simulink library "tqd"  (R2021b)
settings: Solver=VariableStepAuto  StartTime=0.0  StopTime=10.0  RelTol=1e-3
undefined symbols (not defined in the file or in its folder): ATQD_APSDecReq_X_kph, ATQD_APSDecReq_Y_mps2, ATQD_APSDecReqCMD_X_kph, ATQD_APSDecReqTs_X_pct, ATQD_APSDecTimeGain_X_Deg, ATQD_APSDecTimeGain_Y_s, ATQD_APSReqLowSpd_X_Deg, ATQD_AutoHoldReleaseBPS_X_Deg, ATQD_AWDLoadTrqnsGain_X_kg, ATQD_AWDLoadTrqnsGain_Y_pct, ATQD_BOSEnBPSPosn_X_kph, ATQD_BOSMap_X_rpm, ATQD_BOSMap_Y_pct, ATQD_CreepBaseTqD_X_kph, ATQD_CreepBaseTqD_Y_Deg, ATQD_CreepBaseTqR_X_kph, ATQD_CreepBaseTqR_Y_Deg, ATQD_CreepBPSDisPosn_X_Deg, ATQD_CreepBPSDisPosnR_X_Deg, ATQD_CreepBPSEnPosn_X_Deg, ATQD_CreepBPSEnPosnR_X_Deg, ATQD_CreepDeltaTq_X_kph, ATQD_CreepIterm_X_kph, ATQD_CreepIterm_Y_kph, ATQD_CreepItermMaxLimit_X_pct, ATQD_CreepPreloadTime_X_kph, ATQD_CreepPreloadTq_X_kph, ATQD_CreepPreloadTq_Y_s, ATQD_CreepProtTq_X_Deg, ATQD_CreepPterm_X_kph, ATQD_ECOTqMapD_X_rpm, ATQD_ECOTqMapD_Y_pct, ATQD_EOPDTqMapDCon_X_rpm, ATQD_EOPDTqMapDCon_Y_Deg, ATQD_EstInitVehWeight_X_c, ATQD_LHMRollGenMapD_X_rpm, ATQD_LHMRollGenMapD_Y_rpm, ATQD_LHMTqMapD_X_rpm, ATQD_LHMTqMapD_Y_pct, ATQD_NL1TqMapD_X_rpm, ATQD_NL1TqMapD_Y_pct, ATQD_NOPDTqMapDCon_X_rpm, ATQD_NOPDTqMapDCon_Y_Deg, ATQD_NRMRrEDUSpRat_X_rpm, ATQD_NRMRrEDUSpRat_Y_Nm, ATQD_OPDHoldDownRelDelay_X_Deg, ATQD_OPDHoldEnSpd_X_Deg, ATQD_OPDHoldRelDetTime_X_Deg, ATQD_OPDHoldReleaseTq_X_Deg, ATQD_OrigPedTqLowLim_X_Deg, ATQD_OrigPedTqLowLim_Y_pct, ATQD_PedalMapClimbUpLim_X_rpm, ATQD_PedalMapClimbUpLim_Y_Deg, ATQD_PreLoadTq_X_s, ATQD_RollGenMapEL1_X_rpm, ATQD_RollGenMapEL1_Y_rpm, ATQD_SL1TqMapD_X_rpm, ATQD_SL1TqMapD_Y_pct, ATQD_SlideRegenTqGain_X_Gps, ATQD_SlideRegenTqGain_Y_pct ... (+444)
libraries: hcu_lib x70, simulink x61, tqr x1
(part 6 of 14)

== system tqd/TQD/TorqueDemand/Signal_convert/RWDMCUReadyExt_flg ==
  VINP_RrMCUErr_enum : Inport
  Action Port : ActionPort
  Constant : Constant  Value=ENUM_MCUWARN_LV0
  Constant1 : Constant  Value=ENUM_MCUWARN_NOERROR
  Equal : RelationalOperator  Operator===  OutDataTypeStr=boolean  RndMeth=Simplest
  Equal1 : RelationalOperator  Operator===  OutDataTypeStr=boolean  RndMeth=Simplest
  Logical Operator : Logic  Operator=OR  AllPortsSameDT=off  OutDataTypeStr=boolean
  VTQD_RWDMCUReadyExt_flg : Outport
  wires:
  Logical Operator/1 -> VTQD_RWDMCUReadyExt_flg/1
  VINP_RrMCUErr_enum/1 -> Equal1/1, Equal/1
  Equal1/1 -> Logical Operator/2
  Equal/1 -> Logical Operator/1
  Constant1/1 -> Equal1/2
  Constant/1 -> Equal/2

== system tqd/TQD/TorqueDemand/Signal_convert/Regen Level Switch Botton ==
  task_time_s : Inport
  SWC_RegenUp : Inport  Port=2
  SWC_RegenDown : Inport  Port=3
  Constant13 : Constant  Value=ENUM_REGENSWSTA_SHORTPRESSUP
  Constant18 : Constant  Value=ENUM_REGENSWSTA_LONGPRESSUP
  Constant21 : Constant  Value=ENUM_REGENSWSTA_SHORTPRESSDOWN
  Constant23 : Constant  Value=ENUM_REGENSWSTA_LONGPRESSDOWN
  Constant24 : Constant  Value=ENUM_REGENSWSTA_NOACTION
  RegenDOWN : Subsystem
  RegenUP : Subsystem
  Switch{4,6..8} (4 alike) : Switch  Criteria=u2 ~= 0
  VTQD_RegenSWSta_enum : Outport
  wires:
  [SWC_RegenUP] -> RegenUP/2(SWC_RegenUp)
  Constant24/1 -> Switch8/3
  Constant13/1 -> Switch4/1
  [SWC_RegenDown] -> RegenDOWN/3(SWC_RegenDOWN)
  RegenDOWN/2(VTQD_RegenDownLongP_flg) -> Switch8/2
  Constant23/1 -> Switch8/1
  Constant21/1 -> Switch7/1
  Switch7/1 -> Switch6/3
  RegenDOWN/1(SWC_RegenDownShort_flg) -> Switch7/2
  [SWC_RegenUP] -> RegenDOWN/2(SWC_RegenUp)
  Constant18/1 -> Switch6/1
  RegenUP/2(VTQD_RegenUpLongP_flg) -> Switch6/2
  Switch6/1 -> Switch4/3
  RegenUP/1(SWC_RegenUpShort_flg) -> Switch4/2
  [SWC_RegenDown] -> RegenUP/3(SWC_RegenDOWN)
  SWC_RegenUp/1 -> [SWC_RegenUP]
  SWC_RegenDown/1 -> [SWC_RegenDown]
  Switch8/1 -> Switch7/3
  Switch4/1 -> VTQD_RegenSWSta_enum/1
  task_time_s/1 -> [task_time_s]
  [task_time_s] -> RegenUP/1(task_time_s)
  [task_time_s] -> RegenDOWN/1(task_time_s)

== system tqd/TQD/TorqueDemand/Signal_convert/SpdCtrlBotton Behavior ==
  note: If press time more then Long press's limit then go Long press only. Else go short press only. Else if no press.
  note: Long press or Short press
  SWC_ACC_Sta : Inport
  TASK_TIME : Inport  Port=2
  AND : Logic  AllPortsSameDT=off  OutDataTypeStr=boolean
  Constant10 : Constant  Value=FALSE
  Constant3 : Constant  Value=KTQD_SpdModeShortPLim_s
  Constant7 : Constant  Value=FALSE
  Default 3 sec : Constant  Value=KTQD_SpdModeLongPLim_s
  DelayEnable_LONG_PRESS : hcu_lib/Basic_Blocks/DelayEnable
  DelayEnable_SHORT_PRESS : hcu_lib/Basic_Blocks/DelayEnable
  Detect Decrease1 : simulink/Logic and Bit Operations/Detect Decrease  vinit=0.0  OutDataTypeStr=boolean
  Detect Decrease2 : simulink/Logic and Bit Operations/Detect Decrease  vinit=0.0  OutDataTypeStr=boolean
  Detect Increase : simulink/Logic and Bit Operations/Detect Increase  vinit=0.0  OutDataTypeStr=boolean
  Switch1 : Switch  Criteria=u2 > Threshold
  Switch2 : Switch  Criteria=u2 ~= 0
  VTQD_SpdCtrlShortP_flg : Outport
  "VTQD_SpdCtrlLongP_flg\t" : Outport  Port=2
  wires:
  Detect Increase/1 -> "VTQD_SpdCtrlLongP_flg\t"/1
  [TASK_TIME] -> DelayEnable_LONG_PRESS/3
  Default 3 sec/1 -> DelayEnable_LONG_PRESS/2
  [TASK_TIME] -> DelayEnable_SHORT_PRESS/3
  Constant3/1 -> DelayEnable_SHORT_PRESS/2
  DelayEnable_SHORT_PRESS/1 -> Detect Decrease2/1
  Constant7/1 -> Switch1/3
  DelayEnable_LONG_PRESS/1 -> Switch1/1, Switch1/2
  [Short_press_falling_Edge] -> AND/1
  [Long_press] -> Detect Decrease1/1, Detect Increase/1
  Constant10/1 -> Switch2/1
  [Short_press_falling_Edge] -> Switch2/3
  [SWC_ACC_Sta] -> DelayEnable_SHORT_PRESS/1, DelayEnable_LONG_PRESS/1
  AND/1 -> Switch2/2
  Switch2/1 -> VTQD_SpdCtrlShortP_flg/1
  SWC_ACC_Sta/1 -> [SWC_ACC_Sta]
  Detect Decrease1/1 -> AND/2
  Detect Decrease2/1 -> [Short_press_falling_Edge]
  Switch1/1 -> [Long_press]
  TASK_TIME/1 -> [TASK_TIME]

== system tqd/TQD/TorqueDemand/Signal_convert/Speed Setting Mode ==
  note: Botton logic
  note: INPUT Signal
  note: PWRSTA and DRIVE GEAR GOOD
  note: OUTPUT SET SPEED
  VPMM_PowerSta_enum : Inport
  VTQD_ShiftGearPosn_enum : Inport  Port=2
  VINP_VehSpeed_kph : Inport  Port=3
  VTQD_SpdCtrlMode_enum : Inport  Port=4
  VINP_ADASACCSta_enum : Inport  Port=5
  VVMC_CCCtrlSta_enum : Inport  Port=6
  VVMC_MSACtrlSta_enum : Inport  Port=7
  VINP_ADASVehSpdLim_kph : Inport  Port=8
  VTQD_SWCResUpSta_flg : Inport  Port=9
  VTQD_SWCSetDownSta_flg : Inport  Port=10
  VTQD_SWCCancelSta_flg : Inport  Port=11
  task_time_s : Inport  Port=12
  VVMC_LVDAACCStatusInformation_flg : Inport  Port=13
  VVMC_ACCObjDist_m : Inport  Port=14
  VVMC_MeterIndSpeed_raw32 : Inport  Port=15
  VINP_Distanceunit_flg : Inport  Port=16
  ACC Speed Setting ON : Subsystem  TreatAsAtomicUnit=on
  AND{1..5} (5 alike) : Logic  AllPortsSameDT=off  OutDataTypeStr=boolean
  CC Speed Setting ON : Subsystem  TreatAsAtomicUnit=on
  Constant : Constant  Value=ZERO_INT
  Constant1 : Constant  Value=ENUM_SPDCTRLMODE_CC
  Constant10 : Constant  Value=ENUM_SPDCTRLMODE_ISA
  Constant11 : Constant  Value=ENUM_SPDCTRLMODE_OFF
  Constant12 : Constant  Value=KTQD_SetSpdDeltaLongFit_kph
  Constant13 : Constant  Value=ZERO_INT
  Constant2 : Constant  Value=ENUM_POWERSTA_READY
  Constant3 : Constant  Value=ENUM_SPDCTRLMODE_ACC
  Constant4 : Constant  Value=ENUM_GEARPOSNTOCAN_D
  Constant5 : Constant  Value=ENUM_SPDCTRLMODE_MSA
  Constant6 : Constant  Value=ENUM_SPDCTRLMODE_ISA
  Constant7 : Constant  Value=ENUM_SPDCTRLMODE_ACC
  Constant8 : Constant  Value=ENUM_SPDCTRLMODE_CC
  Constant9 : Constant  Value=ENUM_SPDCTRLMODE_MSA
  Data Type Conversion : DataTypeConversion  OutDataTypeStr=uint8
  Delay : Delay  DelayLength=1
  Else Speed Setting On : Subsystem  TreatAsAtomicUnit=on
  Equal{1..11} (11 alike) : RelationalOperator  Operator===  OutDataTypeStr=boolean  RndMeth=Simplest
  ISA Speed Setting ON : Subsystem  TreatAsAtomicUnit=on
  If : If  NumInputs=4  IfExpression=u1 ~= 0  ElseIfExpressions=u2 ~= 0, u3~= 0, u4~= 0
  MSA Speed Setting ON : Subsystem  TreatAsAtomicUnit=on
  Rem : Math  Operator=rem  SaturateOnIntegerOverflow=on
  Switch{,1..4} (5 alike) : Switch  Criteria=u2 ~= 0
  VTQD_SWCCancelP_flg : Subsystem
  VTQD_SWCResUpPress_enum : Subsystem
  VTQD_SWCSetDownPress_enum : Subsystem
  VTQD_SetSpd_kph : Outport
  wires:
  MSA Speed Setting ON/1(VSCP_MSASetSpd_kph) -> [VTQD_MSASetSpd_kph]  "VTQD_MSASetSpd_kph"
  CC Speed Setting ON/1(VTQD_CCSetSpd_kph) -> [VTQD_CCSetSpd_kph]  "VTQD_CCSetSpd_kph"
  VVMC_CCCtrlSta_enum/1 -> [VVMC_CCCtrlSta_enum]
  VINP_ADASVehSpdLim_kph/1 -> [VINP_ADASVehSpdLim_kph]
  task_time_s/1 -> [task_time_s]
  Switch/1 -> [VTQD_SetSpd_kph], VTQD_SetSpd_kph/1
  Constant/1 -> Switch4/1
  Switch4/1 -> Switch3/3
  Equal11/1 -> Switch4/2
  [VTQD_SpdCtrlMode_enum] -> Equal11/1
  Constant11/1 -> Equal11/2
  Switch3/1 -> Switch2/3
  Constant10/1 -> Equal10/2
  [VTQD_SpdCtrlMode_enum] -> Equal10/1
  Equal10/1 -> Switch3/2
  [VTQD_ISASetSpd_kph] -> Switch3/1
  Switch2/1 -> Switch1/3
  [VTQD_MSASetSpd_kph] -> Switch2/1
  Equal9/1 -> Switch2/2
  [VTQD_SpdCtrlMode_enum] -> Equal9/1
  Constant9/1 -> Equal9/2
  Switch1/1 -> Switch/3
  Constant8/1 -> Equal8/2
  [VTQD_SpdCtrlMode_enum] -> Equal8/1
  Equal8/1 -> Switch1/2
  [VTQD_CCSetSpd_kph] -> Switch1/1
  [VTQD_ACCSetSpd_kph] -> Switch/1
  Equal7/1 -> Switch/2
  [VTQD_SpdCtrlMode_enum] -> Equal7/1
  Constant7/1 -> Equal7/2
  ISA Speed Setting ON/1(VTQD_ISASetSpd_kph) -> [VTQD_ISASetSpd_kph]  "VTQD_ISASetSpd_kph"
  If/5 -> Else Speed Setting On/Action
  If/4 -> ISA Speed Setting ON/Action
  AND5/1 -> If/4
  [VTQD_PwrstaANDGearGOOD_flg] -> AND5/1
  [VTQD_SpdCtrlMode_enum] -> Equal6/1
  Constant6/1 -> Equal6/2
  Equal6/1 -> AND5/2
  VVMC_MSACtrlSta_enum/1 -> [VVMC_MSACtrlSta_enum]
  AND4/1 -> If/3
  Equal5/1 -> AND4/2
  Constant5/1 -> Equal5/2
  [VTQD_SpdCtrlMode_enum] -> Equal5/1
  [VTQD_PwrstaANDGearGOOD_flg] -> AND4/1
  If/3 -> MSA Speed Setting ON/Action
  [VVMC_MSACtrlSta_enum] -> MSA Speed Setting ON/1(VVMC_MSACrlSta_enum)
  If/2 -> CC Speed Setting ON/Action
  [VTQD_SWCSetDownPress_enum] -> CC Speed Setting ON/3("VTQD_SWCSetDownPress_enum  ")
  [VTQD_SWCResUpPress_enum] -> CC Speed Setting ON/2("VTQD_SWCResUpPress_enum  ")
  [VVMC_CCCtrlSta_enum] -> CC Speed Setting ON/1(VVMC_CCCtrlSta_enum)
  VTQD_SWCCancelSta_flg/1 -> [VTQD_SWCCancelSta_flg]
  VINP_ADASACCSta_enum/1 -> [VINP_ADASACCSta_enum]
  VINP_VehSpeed_kph/1 -> [VINP_VehSpeed_kph]
  VTQD_SWCSetDownSta_flg/1 -> [VTQD_SWCSetDownSta_flg]
  VTQD_SWCResUpSta_flg/1 -> [VTQD_SWCResUpSta_flg]
  AND3/1 -> If/2
  [VTQD_PwrstaANDGearGOOD_flg] -> AND3/1
  [VTQD_SpdCtrlMode_enum] -> Equal1/1
  Constant1/1 -> Equal1/2
  Equal1/1 -> AND3/2
  AND2/1 -> [VTQD_PwrstaANDGearGOOD_flg]
  [VPMM_PowerSta_enum] -> Equal2/1
  Constant2/1 -> Equal2/2
  [VTQD_ShiftGearPosn_enum] -> Equal4/1
  Constant4/1 -> Equal4/2
  Equal2/1 -> AND2/1
  Equal4/1 -> AND2/2
  AND1/1 -> If/1
  Equal3/1 -> AND1/2
  Constant3/1 -> Equal3/2
  [VTQD_SpdCtrlMode_enum] -> Equal3/1
  If/1 -> ACC Speed Setting ON/Action
  VTQD_SpdCtrlMode_enum/1 -> [VTQD_SpdCtrlMode_enum]
  [VTQD_PwrstaANDGearGOOD_flg] -> AND1/1
  VTQD_ShiftGearPosn_enum/1 -> [VTQD_ShiftGearPosn_enum]
  VPMM_PowerSta_enum/1 -> [VPMM_PowerSta_enum]
  [VINP_ADASVehSpdLim_kph] -> ISA Speed Setting ON/1(VINP_ADASVehSpdLim_kph)
  [VTQD_SWCResUpSta_flg] -> VTQD_SWCResUpPress_enum/1(INPUT)
  VTQD_SWCResUpPress_enum/1(OUTPUT) -> [VTQD_SWCResUpPress_enum]  "VTQD_SWCResUpPress_enum"
  [task_time_s] -> VTQD_SWCSetDownPress_enum/2(task_time_s)
  [VTQD_SWCSetDownSta_flg] -> VTQD_SWCSetDownPress_enum/1(INPUT)
  VTQD_SWCSetDownPress_enum/1(OUTPUT) -> [VTQD_SWCSetDownPress_enum]  "VTQD_SWCSetDownPress_enum"
  [task_time_s] -> VTQD_SWCResUpPress_enum/2(task_time_s)
  VTQD_SWCCancelP_flg/1(Falling_edge) -> [VTQD_SWCCancelP_flg]  "VTQD_SWCCancelP_flg"
  [VTQD_SWCCancelSta_flg] -> VTQD_SWCCancelP_flg/1(INPUT)
  [VTQD_SWCResUpPress_enum] -> MSA Speed Setting ON/2("VTQD_SWCResUpPress_enum  ")
  [VTQD_SWCSetDownPress_enum] -> MSA Speed Setting ON/3("VTQD_SWCSetDownPress_enum  ")
  Rem/1 -> Data Type Conversion/1
  Data Type Conversion/1 -> [VTQD_SetSpdDeltaLongFit_kph]  "VTQD_SetSpdDeltaLongFit_kph"
  [VTQD_SetSpd_kph] -> Delay/1
  Delay/1 -> Rem/1
  Constant12/1 -> Rem/2
  [VTQD_SetSpdDeltaLongFit_kph] -> CC Speed Setting ON/5(VTQD_SetSpdDeltaLongFit_kph)
  [VVMC_MeterIndSpeed_raw32] -> CC Speed Setting ON/4(VVMC_MeterIndSpeed_raw32)
  [VVMC_MeterIndSpeed_raw32] -> MSA Speed Setting ON/4(VVMC_MeterIndSpeed_raw32)
  [VTQD_SetSpdDeltaLongFit_kph] -> MSA Speed Setting ON/5(VTQD_SetSpdDeltaLongFit_kph)
  Constant13/1 -> Else Speed Setting On/1(In)
  Else Speed Setting On/1(Out) -> [VTQD_ElseSetSpd_kph]
  [VTQD_ElseSetSpd_kph] -> Switch4/3
  [VINP_ADASACCSta_enum] -> ACC Speed Setting ON/7(VINP_ADASACCSta_enum)
  [VTQD_SWCResUpSta_flg] -> ACC Speed Setting ON/1(VTQD_SWCResUpSta_flg)
  VVMC_ACCObjDist_m/1 -> ACC Speed Setting ON/5(VVMC_ACCObjDist_m)
  [VTQD_SWCSetDownSta_flg] -> ACC Speed Setting ON/2(VTQD_SWCSetDownSta_flg)
  [VVMC_MeterIndSpeed_raw32] -> ACC Speed Setting ON/6(VVMC_MeterIndSpeed_raw32)
  [task_time_s] -> ACC Speed Setting ON/3(task_time_s)
  ACC Speed Setting ON/1(VTQD_ACCSetSpd_kph) -> [VTQD_ACCSetSpd_kph]  "VTQD_ACCSetSpd_kph"
  VVMC_LVDAACCStatusInformation_flg/1 -> ACC Speed Setting ON/4(VVMC_LVDAACCStatusInformation_flg)
  VVMC_MeterIndSpeed_raw32/1 -> [VVMC_MeterIndSpeed_raw32]
  VINP_Distanceunit_flg/1 -> [VINP_Distanceunit_flg]
  [VINP_Distanceunit_flg] -> ACC Speed Setting ON/8(VINP_Distanceunit_flg)
  [VINP_Distanceunit_flg] -> CC Speed Setting ON/6(VINP_Distanceunit_flg)
  [VINP_Distanceunit_flg] -> MSA Speed Setting ON/6(VINP_Distanceunit_flg)

== system tqd/TQD/TorqueDemand/Signal_convert/VTQD_IVIISAOffsetSpdCHOOSE_flg ==
  VTQD_IVIISAOffsetSpd_enum : Inport
  Constant : Constant  Value=ENUM_IVIISAOFFSETSPD_MIUNS10KPH
  Constant1 : Constant  Value=ENUM_IVIISAOFFSETSPD_MIUNS5KPH
  Constant2 : Constant  Value=ENUM_IVIISAOFFSETSPD_0KPH
  Constant3 : Constant  Value=ENUM_IVIISAOFFSETSPD_PLUS5KPH
  Constant4 : Constant  Value=ENUM_IVIISAOFFSETSPD_PLUS10KPH
  Constant5 : Constant  Value=ENUM_IVIISAOFFSETSPD_MIUNS5MPH
  Constant6 : Constant  Value=ENUM_IVIISAOFFSETSPD_0MPH
  Constant7 : Constant  Value=ENUM_IVIISAOFFSETSPD_PLUS5MPH
  Constant8 : Constant  Value=TRUE
  Constant9 : Constant  Value=FALSE
  Equal{,1..7} (8 alike) : RelationalOperator  Operator===  OutDataTypeStr=boolean  RndMeth=Simplest
  OR : Logic  Operator=OR  Inputs=8  AllPortsSameDT=off  OutDataTypeStr=boolean
  Switch : Switch  Criteria=u2 ~= 0
  VTQD_IVIISAOffsetSpdCHOOSE_flg : Outport
  wires:
  VTQD_IVIISAOffsetSpd_enum/1 -> [VTQD_IVIISAOffsetSpd_enum], Equal/1
  Constant/1 -> Equal/2
  Equal/1 -> OR/1
  Constant1/1 -> Equal1/2
  Equal1/1 -> OR/2
  Equal2/1 -> OR/3
  Constant2/1 -> Equal2/2
  Constant5/1 -> Equal5/2
  Equal5/1 -> OR/6
  Equal4/1 -> OR/5
  Constant4/1 -> Equal4/2
  Equal3/1 -> OR/4
  Constant3/1 -> Equal3/2
  Equal6/1 -> OR/7
  Constant6/1 -> Equal6/2
  Constant7/1 -> Equal7/2
  Equal7/1 -> OR/8
  OR/1 -> Switch/2
  Constant8/1 -> Switch/1
  Constant9/1 -> Switch/3
  Switch/1 -> VTQD_IVIISAOffsetSpdCHOOSE_flg/1  "VTQD_IVIISAOffsetSpdCHOOSE_flg"
  [VTQD_IVIISAOffsetSpd_enum] -> Equal1/1
  [VTQD_IVIISAOffsetSpd_enum] -> Equal2/1
  [VTQD_IVIISAOffsetSpd_enum] -> Equal4/1
  [VTQD_IVIISAOffsetSpd_enum] -> Equal6/1
  [VTQD_IVIISAOffsetSpd_enum] -> Equal5/1
  [VTQD_IVIISAOffsetSpd_enum] -> Equal7/1
  [VTQD_IVIISAOffsetSpd_enum] -> Equal3/1

== system tqd/TQD/TorqueDemand/Signal_convert/VehWeightEst ==
  VTQD_AfterAvailableTqDemRr_Nm : Inport
  VTQR_NoABSREDUWhlTqReq_Nm : Inport  Port=2
  VTQR_NoABSFEDUWhlTqReq_Nm : Inport  Port=3
  VTQD_AfterAvailableTqDemFr_Nm : Inport  Port=4
  VTQD_GearActualPosn_enum : Inport  Port=5
  VINP_VehSpeed_kph : Inport  Port=6
  VTQD_RollRegenDisableReq_flg : Inport  Port=7
  VINP_RegenMode_enum : Inport  Port=8
  VTQD_LowIdleAccPedal_flg : Inport  Port=9
  VTQD_BrkSwSta_flg : Inport  Port=10
  VINP_RrRBCActive_flg : Inport  Port=11
  VINP_FrRBCActive_flg : Inport  Port=12
  VINP_GRADE_Deg : Inport  Port=13
  task_time_s : Inport  Port=14
  VVMC_LongAcc_Gps : Inport  Port=15
  VINP_FrEDURealTMTq_Nm : Inport  Port=16
  VINP_RrEDURealTMTq_Nm : Inport  Port=17
  VINP_DriverSeatBeltCmd_flg : Inport  Port=18
  VINP_PsngrSeatBeltCmd_flg : Inport  Port=19
  VINP_RDriverSeatBeltCmd_flg : Inport  Port=20
  VINP_RCenterSeatBeltCmd_flg : Inport  Port=21
  VINP_RPsngrSeatBeltCmd_flg : Inport  Port=22
  Calaulation : Subsystem
  Condition : Subsystem
  Desicion : Subsystem
  VTQD_EstVehWeightResult_kg : Outport
  wires:
  Calaulation/2(VTQD_EstFrRealTqCheckPass_flg) -> [VTQD_EstFrRealTqCheckPass_flg]
  [VTQD_BrkSwSta_flg] -> Condition/10(VTQD_BrkSwSta_flg)
  Condition/2(VTQD_VehWeightEstDis_flg) -> [VTQD_VehWeightEstDis_flg]
  VTQD_RollRegenDisableReq_flg/1 -> [VTQD_RollRegenDisableReq_flg]
  [VINP_VehSpeed_kph] -> Calaulation/8(VINP_VehSpeed_kph)
  [VINP_PsngrSeatBeltCmd_flg] -> Desicion/5(VINP_PsngrSeatBeltCmd_flg)
  VTQD_BrkSwSta_flg/1 -> [VTQD_BrkSwSta_flg]
  [task_time_s] -> Calaulation/1(task_time_s)
  [VINP_RCenterSeatBeltCmd_flg] -> Desicion/7(VINP_RCenterSeatBeltCmd_flg)
  [VINP_FrEDURealTMTq_Nm] -> Calaulation/6(VINP_FrEDURealTMTq_Nm)
  VINP_RrEDURealTMTq_Nm/1 -> [VINP_RrEDURealTMTq_Nm]
  [VTQD_VehWeightEstEnd_flg] -> Calaulation/4(VTQD_VehWeightEstEnd_flg)
  [VTQR_NoABSREDUWhlTqReq_Nm] -> Condition/2(VTQR_NoABSREDUWhlTqReq_Nm)
  [VTQD_VehWeightEstDis_flg] -> Calaulation/3(VTQD_VehWeightEstDis_flg)
  [VVMC_LongAcc_Gps] -> Calaulation/5(VVMC_LongAcc_Gps)
  VTQD_GearActualPosn_enum/1 -> [VTQD_GearActualPosn_enum]
  [VTQD_EstRrRealTqCheckPass_flg] -> Desicion/11(VTQD_EstRrRealTqCheckPass_flg)
  VINP_RCenterSeatBeltCmd_flg/1 -> [VINP_RCenterSeatBeltCmd_flg]
  [VTQD_EstVehWeightResult_kg] -> VTQD_EstVehWeightResult_kg/1
  [VTQD_RollRegenDisableReq_flg] -> Condition/7(VTQD_RollRegenDisableReq_flg)
  [VINP_RPsngrSeatBeltCmd_flg] -> Desicion/8(VINP_RPsngrSeatBeltCmd_flg)
  [VTQD_VehWeightEstEn_flg] -> Calaulation/2(VTQD_VehWeightEstEn_flg)
  VINP_GRADE_Deg/1 -> [VINP_GRADE_Deg]
  VTQD_AfterAvailableTqDemRr_Nm/1 -> [VTQD_AfterAvailableTqDemRr_Nm]
  [VINP_RegenMode_enum] -> Condition/8(VINP_RegenMode_enum)
  task_time_s/1 -> [task_time_s]
  [VTQD_EstLongAccCheckPass_flg] -> Desicion/9(VTQD_EstLongAccCheckPass_flg)
  [VTQD_LowIdleAccPedal_flg] -> Condition/9(VTQD_LowIdleAccPedal_flg)
  VINP_RPsngrSeatBeltCmd_flg/1 -> [VINP_RPsngrSeatBeltCmd_flg]
  [VTQD_GearActualPosn_enum] -> Condition/5(VTQD_GearActualPosn_enum)
  [VINP_RrRBCActive_flg] -> Condition/11(VINP_RrRBCActive_flg)
  Condition/1(VTQD_VehWeightEstEn_flg) -> [VTQD_VehWeightEstEn_flg]
  Desicion/1(VTQD_VehWeightEstEnd_flg) -> [VTQD_VehWeightEstEnd_flg]
  [VINP_DriverSeatBeltCmd_flg] -> Desicion/4(VINP_DriverSeatBeltCmd_flg)
  [VTQD_VehWeightEstDis_flg] -> Desicion/2(VTQD_VehWeightEstDis_flg)
  VINP_DriverSeatBeltCmd_flg/1 -> [VINP_DriverSeatBeltCmd_flg]
  VINP_VehSpeed_kph/1 -> [VINP_VehSpeed_kph]
  [task_time_s] -> Condition/14(task_time_s)
  VTQR_NoABSREDUWhlTqReq_Nm/1 -> [VTQR_NoABSREDUWhlTqReq_Nm]
  [VINP_RrEDURealTMTq_Nm] -> Calaulation/7(VINP_RrEDURealTMTq_Nm)
  [VTQR_NoABSFEDUWhlTqReq_Nm] -> Condition/3(VTQR_NoABSFEDUWhlTqReq_Nm)
  [VTQD_AfterAvailableTqDemFr_Nm] -> Condition/4(VTQD_AfterAvailableTqDemFr_Nm)
  VINP_RrRBCActive_flg/1 -> [VINP_RrRBCActive_flg]
  [VINP_FrRBCActive_flg] -> Condition/12(VINP_FrRBCActive_flg)
  VTQD_AfterAvailableTqDemFr_Nm/1 -> [VTQD_AfterAvailableTqDemFr_Nm]
  VINP_FrEDURealTMTq_Nm/1 -> [VINP_FrEDURealTMTq_Nm]
  VTQD_LowIdleAccPedal_flg/1 -> [VTQD_LowIdleAccPedal_flg]
  [VTQD_AfterAvailableTqDemRr_Nm] -> Condition/1(VTQD_AfterAvailableTqDemRr_Nm)
  [VINP_GRADE_Deg] -> Condition/13(VINP_GRADE_Deg)
  [VINP_VehSpeed_kph] -> Condition/6(VINP_VehSpeed_kph)
  VINP_RegenMode_enum/1 -> [VINP_RegenMode_enum]
  VTQR_NoABSFEDUWhlTqReq_Nm/1 -> [VTQR_NoABSFEDUWhlTqReq_Nm]
  VINP_RDriverSeatBeltCmd_flg/1 -> [VINP_RDriverSeatBeltCmd_flg]
  VINP_PsngrSeatBeltCmd_flg/1 -> [VINP_PsngrSeatBeltCmd_flg]
  Calaulation/3(VTQD_EstRrRealTqCheckPass_flg) -> [VTQD_EstRrRealTqCheckPass_flg]
  [VTQD_EstFrRealTqCheckPass_flg] -> Desicion/10(VTQD_EstFrRealTqCheckPass_flg)
  Calaulation/1(VTQD_EstLongAccCheckPass_flg) -> [VTQD_EstLongAccCheckPass_flg]
  VVMC_LongAcc_Gps/1 -> [VVMC_LongAcc_Gps]
  [VTQD_VehWeightEstEnd_flg] -> Condition/15(VTQD_VehWeightEstEnd_flg)
  [VINP_RDriverSeatBeltCmd_flg] -> Desicion/6(VINP_RDriverSeatBeltCmd_flg)
  [VTQD_EstVehWeight_kg] -> Desicion/3(VTQD_EstVehWeight_kg)
  Calaulation/4(VTQD_EstVehWeight_kg) -> [VTQD_EstVehWeight_kg]
  Desicion/2(VTQD_EstVehWeightResult_kg) -> [VTQD_EstVehWeightResult_kg]
  [task_time_s] -> Desicion/1(task_time_s)
  VINP_FrRBCActive_flg/1 -> [VINP_FrRBCActive_flg]

== system tqd/TQD/TorqueDemand/Signal_convert/Vehicle to Meter Speed ==
  InputSpeed : Inport
  Add : Sum
  Constant1 : Constant  Value=KTQD_Veh2MetSpdAdd_kph
  Constant11 : Constant  Value=KTQD_Veh2MetSpdGain_c
  Product : Product
  OutputSpeed : Outport
  wires:
  Constant1/1 -> Add/2
  Add/1 -> OutputSpeed/1
  Constant11/1 -> Product/2
  Product/1 -> Add/1
  InputSpeed/1 -> Product/1

== system tqd/TQD/TorqueDemand/TorqueModule/ActualWhTqWithDirection ==
  VTQD_GearActualPosn_enum : Inport
  VTQD_AfterAvailableTqDemF_Nm : Inport  Port=2
  VTQD_AfterAvailableTqDemR_Nm : Inport  Port=3
  Constant1 : Constant  Value=ONE_FLOAT
  Constant2 : Constant  Value=MINUSONE_FLOAT
  Constant5 : Constant  Value=ENUM_GEARACTUALPOSN_R
  Equal : RelationalOperator  Operator===  OutDataTypeStr=boolean  RndMeth=Simplest
  Product : Product
  Product1 : Product
  Switch : Switch  Criteria=u2 ~= 0
      settings: AttributesFormatString=<%<Criteria>>
  VTQD_ActualWhlTqDemF_Nm : Outport
  VTQD_ActualWhlTqDemR_Nm : Outport  Port=2
  wires:
  VTQD_GearActualPosn_enum/1 -> Equal/1
  Constant5/1 -> Equal/2
  Equal/1 -> Switch/2
  VTQD_AfterAvailableTqDemF_Nm/1 -> [VTQD_AfterAvailableTqDemF_Nm]
  VTQD_AfterAvailableTqDemR_Nm/1 -> [VTQD_AfterAvailableTqDemR_Nm]
  Constant2/1 -> Switch/1
  Constant1/1 -> Switch/3
  [VTQD_AfterAvailableTqDemF_Nm] -> Product/1
  Switch/1 -> Product/2, Product1/1
  [VTQD_AfterAvailableTqDemR_Nm] -> Product1/2
  Product/1 -> VTQD_ActualWhlTqDemF_Nm/1  "VTQD_ActualWhlTqDemF_Nm"
  Product1/1 -> VTQD_ActualWhlTqDemR_Nm/1  "VTQD_ActualWhlTqDemR_Nm"

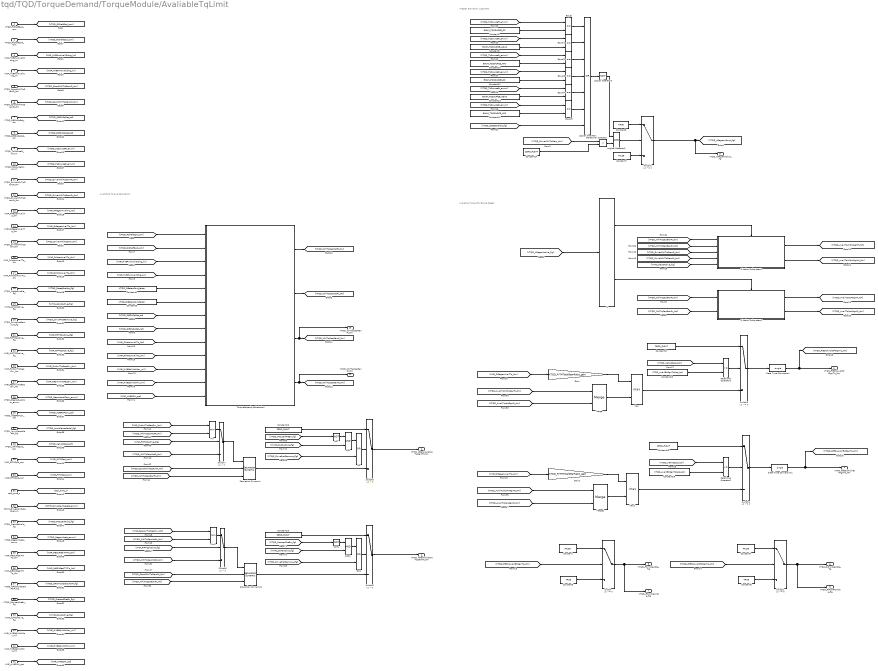
== system tqd/TQD/TorqueDemand/TorqueModule/AvaliableTqLimit ==
  note: Avaiable Torque for B-type Regen
  note: Available Torque Calculation
  note: A-regen activation judgment
  VTQD_FrShaftSpd_rpm : Inport
  VTQD_RrShaftSpd_rpm : Inport  Port=2
  VINP_HVBPwrAvailDchrg_kw : Inport  Port=3
  VINP_HVBPwrAvailChrg_kw : Inport  Port=4
  VTQD_CoordWhlTqDemFr_Nm : Inport  Port=5
  VTQD_CoordWhlTqDemRr_Nm : Inport  Port=6
  VTQD_FrEDUSpRat_rat : Inport  Port=7
  VTQD_RrEDUSpRat_rat : Inport  Port=8
  VTQD_TqSourceFr_enum : Inport  Port=9
  VTQD_TqSourceRr_enum : Inport  Port=10
  VTQD_DriverWhlTqDemFr_Nm : Inport  Port=11
  VTQD_DriverWhlTqDemRr_Nm : Inport  Port=12
  VINP_FrRegenAvailTq_Nm : Inport  Port=13
  VINP_RrRegenAvailTq_Nm : Inport  Port=14
  VTQD_DriverWhlTqDem_Nm : Inport  Port=15
  VINP_FrMotorAvailTq_Nm : Inport  Port=16
  VINP_RrMotorAvailTq_Nm : Inport  Port=17
  VTQD_CreepEnable_flg : Inport  Port=18
  VVMC_ADASActive_flg : Inport  Port=19
  VTQD_DriveProtRemove_flg : Inport  Port=20
  VINP_FrPTCSActive_flg : Inport  Port=21
  VINP_RrPTCSActive_flg : Inport  Port=22
  VINP_FrntAxlTrqReqDrv_Nm : Inport  Port=23
  VINP_RearAxlTrqReqDrv_Nm : Inport  Port=24
  VTQD_GearActualPosn_enum : Inport  Port=25
  VTQD_ActBPSPosn_pct : Inport  Port=26
  VTQD_LowIdleAccPedal_flg : Inport  Port=27
  VTQD_VehActSpd_kph : Inport  Port=28
  VINP_RrTMSpd_rpm : Inport  Port=29
  VINP_FrTMSpd_rpm : Inport  Port=30
  task_time_s : Inport  Port=31
  VPMM_DrivetrainSelect_enum : Inport  Port=32
  VTQD_PreLoadHold_flg : Inport  Port=33
  VTQD_RegenMode_enum : Inport  Port=34
  VINP_FrEDURealTMTq_Nm : Inport  Port=35
  VINP_RrEDURealTMTq_Nm : Inport  Port=36
  VTQD_OPDHoldDelayForP_flg : Inport  Port=37
  VTQD_PreLoadPreEn_flg : Inport  Port=38
  VVMC_CAASActive_flg : Inport  Port=39
  VINP_HVBCellVoltMax_mV : Inport  Port=40
  VINP_HVBCellVoltMin_mV : Inport  Port=41
  VINP_HVBSOH_pct : Inport  Port=42
  AND : Logic  AllPortsSameDT=off  OutDataTypeStr=boolean
  AND1 : Logic  AllPortsSameDT=off  OutDataTypeStr=boolean
  Constant : Constant  Value=FALSE
  Constant1 : Constant  Value=ENUM_TQSOURCE_CC
  Constant10 : Constant  Value=ENUM_TQSOURCE_APS
  Constant11 : Constant  Value=ENUM_TQSOURCE_CC
  Constant12 : Constant  Value=ENUM_TQSOURCE_APS
  Constant13 : Constant  Value=ENUM_TQSOURCE_ADAS
  Constant{14,16..17,19..20} (5 alike) : Constant  Value=ZERO_FLOAT
  Constant15 : Constant  Value=KTQD_AvailBrkRgnTqSpd_kph
  Constant18 : Constant  Value=KTQD_AvailBrkRgnTqSpd_kph
  Constant2 : Constant  Value=KTQD_FrBatapCont_factor
  Constant3 : Constant  Value=TRUE
  Constant4 : Constant  Value=FALSE
  Constant5 : Constant  Value=KTQD_RrBatapCont_factor
  Constant6 : Constant  Value=TRUE
  Constant7 : Constant  Value=FALSE
  Constant8 : Constant  Value=TRUE
  Constant9 : Constant  Value=ENUM_TQSOURCE_ADAS
  Data Type Conversion : DataTypeConversion  OutDataTypeStr=single
  Data Type Conversion1 : DataTypeConversion  OutDataTypeStr=single
  Equal{,1..5} (6 alike) : RelationalOperator  Operator===  OutDataTypeStr=boolean  RndMeth=Simplest
  Gain : Gain  Gain=KTQD_FrTMTotalGearRatio_gain
  Gain1 : Gain  Gain=KTQD_RrTMTotalGearRatio_gain
  If : If  IfExpression=u1 ~= 0
  If Action Subsystem1 : Subsystem  TreatAsAtomicUnit=on
  If Action Subsystem2 : Subsystem  TreatAsAtomicUnit=on
  Logical Operator : Logic  Operator=OR  Inputs=7  AllPortsSameDT=off  OutDataTypeStr=boolean
  Logical Operator1 : Logic  AllPortsSameDT=off  OutDataTypeStr=boolean
  Logical Operator2 : Logic  Operator=NOT  AllPortsSameDT=off  OutDataTypeStr=boolean
  Max : MinMax  Function=max  Inputs=2
  Max1 : MinMax  Function=max  Inputs=2
  Merge : Merge
  Merge1 : Merge
  Min : MinMax  Inputs=2
  Min1 : MinMax  Inputs=2
  NOT : Logic  Operator=NOT  AllPortsSameDT=off  OutDataTypeStr=boolean
  NOT1 : Logic  Operator=NOT  AllPortsSameDT=off  OutDataTypeStr=boolean
  OR : Logic  Operator=OR  AllPortsSameDT=off  OutDataTypeStr=boolean
  OR1 : Logic  Operator=OR  AllPortsSameDT=off  OutDataTypeStr=boolean
  Relational Operator : RelationalOperator  Operator=<  OutDataTypeStr=boolean  RndMeth=Simplest
  Relational Operator1 : RelationalOperator  Operator=<=  OutDataTypeStr=boolean  RndMeth=Simplest
  Relational Operator2 : RelationalOperator  Operator=<=  OutDataTypeStr=boolean  RndMeth=Simplest
  Saturation Dynamic : simulink/Discontinuities/Saturation Dynamic  OutMin=[]  OutMax=[]  OutDataTypeStr=Inherit: Same as second input  OutDataType=fixdt(1, 16)  OutScaling=2^-10  DoSatur=off
  Saturation Dynamic1 : simulink/Discontinuities/Saturation Dynamic  OutMin=[]  OutMax=[]  OutDataTypeStr=Inherit: Same as second input  OutDataType=fixdt(1, 16)  OutScaling=2^-10  DoSatur=off
  Switch : Switch
  Switch1 : Switch
  Switch2 : Switch  Criteria=u2 ~= 0
  Switch3 : Switch  Criteria=u2 ~= 0
  Switch4 : Switch  Criteria=u2 ~= 0
  Switch{5..8} (4 alike) : Switch  Criteria=u2 > Threshold
  TorqueCapacityCalcalation : Subsystem
  VTQD_AfterAvailableTqDemFr_Nm : Outport
  VTQD_AfterAvailableTqDemRr_Nm : Outport  Port=2
  VTQD_FrEDUAvailBrkRgnTq_Nm : Outport  Port=3
  VTQD_RrEDUAvailBrkRgnTq_Nm : Outport  Port=4
  VTQD_FrRgnDecrSta_flg : Outport  Port=5
  VTQD_RrRgnDecrSta_flg : Outport  Port=6
  VTQD_FrRgnPermSta_flg : Outport  Port=7
  VTQD_RrRgnPermSta_flg : Outport  Port=8
  VTQD_ARegenActive_flg : Outport  Port=9
  VTQD_WhlTqCapGenFr_Nm : Outport  Port=10
  VTQD_WhlTqCapGenRr_Nm : Outport  Port=11
  wires:
  VINP_FrRegenAvailTq_Nm/1 -> [VINP_FrRegenAvailTq_Nm]
  VINP_RrRegenAvailTq_Nm/1 -> [VINP_RrRegenAvailTq_Nm]
  Merge1/1 -> Max1/2
  [VINP_RrRegenAvailTq_Nm] -> Gain1/1
  Gain1/1 -> Max1/1
  Gain/1 -> Max/1
  Merge/1 -> Max/2
  [VINP_FrRegenAvailTq_Nm] -> Gain/1
  [VTQD_ARegenActive_flg] -> If/1
  Switch1/1 -> VTQD_RrRgnDecrSta_flg/1, VTQD_RrRgnPermSta_flg/1
  Constant6/1 -> Switch1/3
  Constant4/1 -> Switch1/1
  [VTQD_RrEDUAvailBrkRgnTq_Nm] -> Switch1/2
  Switch/1 -> VTQD_FrRgnDecrSta_flg/1, VTQD_FrRgnPermSta_flg/1
  Constant3/1 -> Switch/3
  Constant/1 -> Switch/1
  [VTQD_FrEDUAvailBrkRgnTq_Nm] -> Switch/2
  If/2 -> If Action Subsystem2/Action
  If/1 -> If Action Subsystem1/Action
  Data Type Conversion1/1 -> VTQD_RrEDUAvailBrkRgnTq_Nm/1, [VTQD_RrEDUAvailBrkRgnTq_Nm]  "VTQD_RrEDUAvailBrkRgnTq_Nm"
  Data Type Conversion/1 -> VTQD_FrEDUAvailBrkRgnTq_Nm/1, [VTQD_FrEDUAvailBrkRgnTq_Nm]  "VTQD_FrEDUAvailBrkRgnTq_Nm"
  TorqueCapacityCalcalation/4(VTQD_WhlTqCapGenRr_Nm) -> VTQD_WhlTqCapGenRr_Nm/1, [VTQD_WhlTqCapGenRr_Nm]
  TorqueCapacityCalcalation/2(VTQD_WhlTqCapMotRr_Nm) -> [VTQD_WhlTqCapMotRr_Nm]
  VTQD_RrShaftSpd_rpm/1 -> [VTQD_RrShaftSpd_rpm]
  [VTQD_RrEDUSpRat_rat] -> TorqueCapacityCalcalation/8(VTQD_RrEDUSpRat_rat)
  [VTQD_FrEDUSpRat_rat] -> TorqueCapacityCalcalation/7(VTQD_FrEDUSpRat_cmd)
  Constant5/1 -> TorqueCapacityCalcalation/6(KTQD_RrBatapCont_factor)
  [VTQD_RrShaftSpd_rpm] -> TorqueCapacityCalcalation/2(VTQD_RrShaftSpd_rpm)
  Constant2/1 -> TorqueCapacityCalcalation/5(KTQD_FrBatapCont_factor)
  [VINP_HVBPwrAvailChrg_kw] -> TorqueCapacityCalcalation/4(VINP_HVBPwrAvailChrg_kw)
  [VINP_HVBPwrAvailDchrg_kw] -> TorqueCapacityCalcalation/3(VINP_HVBPwrAvailDchrg_kw)
  [VTQD_FrShaftSpd_rpm] -> TorqueCapacityCalcalation/1(VTQD_FrShaftSpd_rpm)
  TorqueCapacityCalcalation/1(VTQD_WhlTqCapMotFr_Nm) -> [VTQD_WhlTqCapMotFr_Nm]
  TorqueCapacityCalcalation/3(VTQD_WhlTqCapGenFr_Nm) -> VTQD_WhlTqCapGenFr_Nm/1, [VTQD_WhlTqCapGenFr_Nm]
  If Action Subsystem2/2(VTQD_AvailTqNoARgnRr_Nm) -> [VTQD_AvailTqNoARgnRr_Nm]
  If Action Subsystem2/1(VTQD_AvailTqNoARgnFr_Nm) -> [VTQD_AvailTqNoARgnFr_Nm]
  [VTQD_WhlTqCapGenRr_Nm] -> If Action Subsystem2/2(VTQD_WhlTqCapGenR_Nm)
  [VTQD_WhlTqCapGenFr_Nm] -> If Action Subsystem2/1(VTQD_WhlTqCapGenF_Nm)
  [VTQD_WhlTqCapGenRr_Nm] -> If Action Subsystem1/2(VTQD_WhlTqCapGenR_Nm)
  [VTQD_WhlTqCapGenFr_Nm] -> If Action Subsystem1/1(VTQD_WhlTqCapGenF_Nm)
  [VTQD_DriverWhlTqDemRr_Nm] -> If Action Subsystem1/4(VTQD_DriverWhlTqDemRr_Nm)
  [VTQD_DriverWhlTqDemFr_Nm] -> If Action Subsystem1/3(VTQD_DriverWhlTqDemFr_Nm)
  VTQD_DriverWhlTqDemRr_Nm/1 -> [VTQD_DriverWhlTqDemRr_Nm]
  VTQD_DriverWhlTqDemFr_Nm/1 -> [VTQD_DriverWhlTqDemFr_Nm]
  VTQD_TqSourceFr_enum/1 -> [VTQD_TqSourceFr_enum]
  VTQD_RrEDUSpRat_rat/1 -> [VTQD_RrEDUSpRat_rat]
  VTQD_FrEDUSpRat_rat/1 -> [VTQD_FrEDUSpRat_rat]
  VTQD_CoordWhlTqDemRr_Nm/1 -> [VTQD_CoordWhlTqDemRr_Nm]
  VTQD_CoordWhlTqDemFr_Nm/1 -> [VTQD_CoordWhlTqDemFr_Nm]
  VINP_HVBPwrAvailDchrg_kw/1 -> [VINP_HVBPwrAvailDchrg_kw]
  VTQD_FrShaftSpd_rpm/1 -> [VTQD_FrShaftSpd_rpm]
  VINP_HVBPwrAvailChrg_kw/1 -> [VINP_HVBPwrAvailChrg_kw]
  VTQD_TqSourceRr_enum/1 -> [VTQD_TqSourceRr_enum]
  Switch2/1 -> [VTQD_ARegenActive_flg], VTQD_ARegenActive_flg/1  "VTQD_ARegenActive_flg"
  VTQD_DriverWhlTqDem_Nm/1 -> [VTQD_DriverWhlTqDem_Nm]
  VINP_RrMotorAvailTq_Nm/1 -> [VINP_RrMotorAvailTq_Nm]
  VINP_FrMotorAvailTq_Nm/1 -> [VINP_FrMotorAvailTq_Nm]
  [VINP_FrMotorAvailTq_Nm] -> TorqueCapacityCalcalation/9(VINP_FrMotorAvailTq_Nm)
  [VINP_RrMotorAvailTq_Nm] -> TorqueCapacityCalcalation/10(VINP_RrMotorAvailTq_Nm)
  VTQD_CreepEnable_flg/1 -> [VTQD_CreepEnable_flg]
  [VTQD_TqSourceFr_enum] -> Equal/1
  Constant1/1 -> Equal/2
  Constant9/1 -> Equal1/2
  [VTQD_TqSourceFr_enum] -> Equal1/1
  [VTQD_TqSourceFr_enum] -> Equal2/1
  Constant10/1 -> Equal2/2
  Constant12/1 -> Equal5/2
  [VTQD_TqSourceRr_enum] -> Equal5/1
  [VTQD_TqSourceRr_enum] -> Equal4/1
  Constant13/1 -> Equal4/2
  Constant11/1 -> Equal3/2
  [VTQD_TqSourceRr_enum] -> Equal3/1
  Equal5/1 -> Logical Operator/6
  Equal4/1 -> Logical Operator/5
  Equal3/1 -> Logical Operator/4
  Equal2/1 -> Logical Operator/3
  Equal1/1 -> Logical Operator/2
  Equal/1 -> Logical Operator/1
  [VTQD_CreepEnable_flg] -> Logical Operator/7
  Logical Operator/1 -> Logical Operator2/1
  Logical Operator1/1 -> Switch2/2
  [VTQD_DriverWhlTqDem_Nm] -> Relational Operator/1
  Relational Operator/1 -> Logical Operator1/2
  Constant14/1 -> Relational Operator/2
  Constant7/1 -> Switch2/3
  Constant8/1 -> Switch2/1
  Logical Operator2/1 -> Logical Operator1/1
  Constant17/1 -> Switch3/1
  Relational Operator1/1 -> Switch3/2
  Constant15/1 -> Relational Operator1/2
  Max/1 -> Switch3/3
  Switch3/1 -> Data Type Conversion/1
  Constant20/1 -> Switch4/1
  Max1/1 -> Switch4/3
  Relational Operator2/1 -> Switch4/2
  Constant18/1 -> Relational Operator2/2
  Switch4/1 -> Data Type Conversion1/1
  VVMC_ADASActive_flg/1 -> [VVMC_ADASActive_flg]
  [VVMC_ADASActive_flg] -> If Action Subsystem1/5(VVMC_ADASActive_flg)
  [VTQD_AvailTqNoARgnRr_Nm] -> Merge1/2
  [VTQD_AvailTqWithARgnRr_Nm] -> Merge1/1
  [VTQD_AvailTqNoARgnFr_Nm] -> Merge/2
  [VTQD_AvailTqWithARgnFr_Nm] -> Merge/1
  Constant16/1 -> Switch5/1
  Switch5/1 -> VTQD_AfterAvailableTqDemFr_Nm/1  "VTQD_AfterAvailableTqDemFr_Nm"
  Saturation Dynamic/1 -> Switch5/3
  Constant19/1 -> Switch6/1
  Saturation Dynamic1/1 -> Switch6/3
  Switch6/1 -> VTQD_AfterAvailableTqDemRr_Nm/1  "VTQD_AfterAvailableTqDemRr_Nm"
  VTQD_DriveProtRemove_flg/1 -> [VTQD_DriveProtRemove_flg]
  [VTQD_CoordWhlTqDemFr_Nm] -> Saturation Dynamic/2
  Switch7/1 -> Saturation Dynamic/1  "VTQD_FrAvailableTqUpLimt_Nm"
  [VTQD_WhlTqCapMotFr_Nm] -> Switch7/3
  [VINP_FrPTCSActive_flg] -> Switch7/2
  VINP_RearAxlTrqReqDrv_Nm/1 -> [VINP_RearAxlTrqReqDrv_Nm]
  VINP_FrntAxlTrqReqDrv_Nm/1 -> [VINP_FrntAxlTrqReqDrv_Nm]
  VINP_RrPTCSActive_flg/1 -> [VINP_RrPTCSActive_flg]
  VINP_FrPTCSActive_flg/1 -> [VINP_FrPTCSActive_flg]
  [VINP_RrPTCSActive_flg] -> Switch8/2
  [VTQD_WhlTqCapMotRr_Nm] -> Switch8/3
  Switch8/1 -> Saturation Dynamic1/1  "VTQD_RrAvailableTqUpLimt_Nm"
  [VTQD_CoordWhlTqDemRr_Nm] -> Saturation Dynamic1/2
  [VTQD_WhlTqCapMotFr_Nm] -> Min/2
  Min/1 -> Switch7/1
  [VINP_FrntAxlTrqReqDrv_Nm] -> Min/1
  [VTQD_WhlTqCapMotRr_Nm] -> Min1/2
  Min1/1 -> Switch8/1
  [VINP_RearAxlTrqReqDrv_Nm] -> Min1/1
  VTQD_GearActualPosn_enum/1 -> [VTQD_GearActualPosn_enum]
  VTQD_ActBPSPosn_pct/1 -> [VTQD_ActBPSPosn_pct]
  VTQD_LowIdleAccPedal_flg/1 -> [VTQD_LowIdleAccPedal_flg]
  VTQD_VehActSpd_kph/1 -> [VTQD_VehActSpd_kph]
  VINP_RrTMSpd_rpm/1 -> [VINP_RrTMSpd_rpm]
  VINP_FrTMSpd_rpm/1 -> [VINP_FrTMSpd_rpm]
  task_time_s/1 -> [task_time_s]
  VPMM_DrivetrainSelect_enum/1 -> [VPMM_DrivetrainSelect_enum]
  [VTQD_VehActSpd_kph] -> Relational Operator1/1
  [VTQD_VehActSpd_kph] -> Relational Operator2/1
  [VTQD_WhlTqCapGenFr_Nm] -> Saturation Dynamic/3
  [VTQD_WhlTqCapGenRr_Nm] -> Saturation Dynamic1/3
  VTQD_PreLoadHold_flg/1 -> [VTQD_PreLoadHold_flg]
  VTQD_RegenMode_enum/1 -> [VTQD_RegenMode_enum]
  VINP_RrEDURealTMTq_Nm/1 -> [VINP_RrEDURealTMTq_Nm]
  VINP_FrEDURealTMTq_Nm/1 -> [VINP_FrEDURealTMTq_Nm]
  VTQD_OPDHoldDelayForP_flg/1 -> [VTQD_OPDHoldDelayForP_flg]
  VVMC_CAASActive_flg/1 -> [VVMC_CAASActive_flg]
  VTQD_PreLoadPreEn_flg/1 -> [VTQD_PreLoadPreEn_flg]
  OR/1 -> Switch5/2
  AND/1 -> OR/1
  [VTQD_DriveProtRemove_flg] -> OR/2
  NOT/1 -> AND/1
  [VTQD_PreLoadPreEn_flg] -> NOT/1
  [VVMC_CAASActive_flg] -> AND/2
  NOT1/1 -> AND1/1
  AND1/1 -> OR1/1
  [VVMC_CAASActive_flg] -> AND1/2
  [VTQD_PreLoadPreEn_flg] -> NOT1/1
  [VTQD_DriveProtRemove_flg] -> OR1/2
  OR1/1 -> Switch6/2
  VINP_HVBCellVoltMin_mV/1 -> [VINP_HVBCellVoltMin_mV]
  VINP_HVBSOH_pct/1 -> [VINP_HVBSOH_pct]
  VINP_HVBCellVoltMax_mV/1 -> [VINP_HVBCellVoltMax_mV]
  [VINP_HVBCellVoltMax_mV] -> TorqueCapacityCalcalation/11(VINP_HVBCellVoltMax_mV)
  [VINP_HVBCellVoltMin_mV] -> TorqueCapacityCalcalation/12(VINP_HVBCellVoltMin_mV)
  [VINP_HVBSOH_pct] -> TorqueCapacityCalcalation/13(VINP_HVBSOH_pct)
  If Action Subsystem1/1(VTQD_AvailTqWithARgnFr_Nm) -> [VTQD_AvailTqWithARgnFr_Nm]
  If Action Subsystem1/2(VTQD_AvailTqWithARgnRr_Nm) -> [VTQD_AvailTqWithARgnRr_Nm]

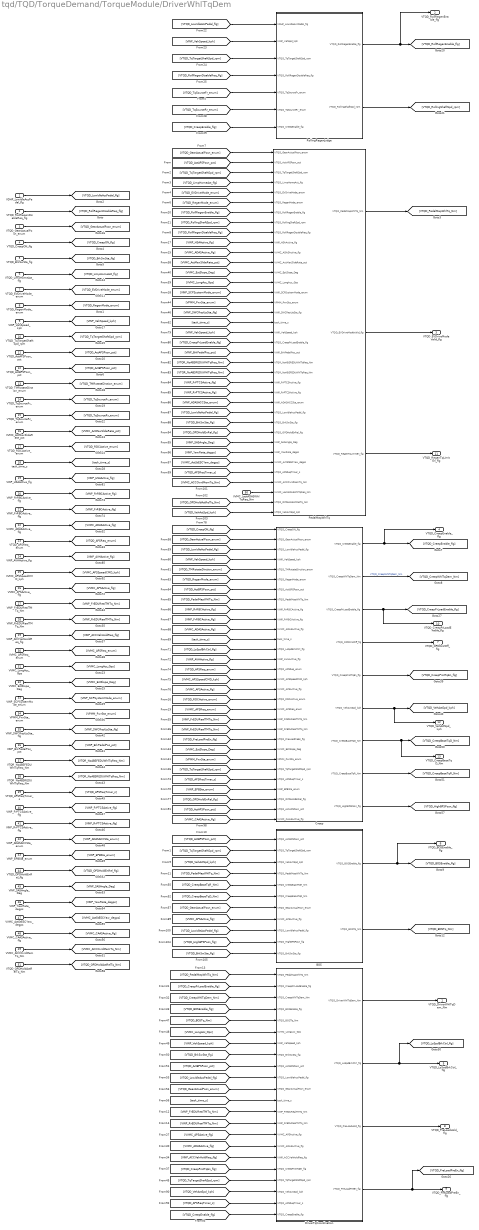
== system tqd/TQD/TorqueDemand/TorqueModule/DriverWhlTqDem ==
  VDHP_LowIdleAccPedal_flg : Inport
  VTQD_RollRegenDisableReq_flg : Inport  Port=2
  VTQD_GearActualPosn_enum : Inport  Port=3
  "VTQD_CreepON_flg " : Inport  Port=4
  VTQD_BrkSwSta_flg : Inport  Port=5
  VTQD_LimpHomeAct_flg : Inport  Port=6
  VTQD_EVDriveMode_enum : Inport  Port=7
  VTQD_RegenMode_enum : Inport  Port=8
  VINP_VehSpeed_kph : Inport  Port=9
  VTQD_TqTargetShaftSpd_rpm : Inport  Port=10
  VTQD_ActAPSPosn_pct : Inport  Port=11
  VTQD_ActBPSPosn_pct : Inport  Port=12
  VTQD_TMRotateDirction_enum : Inport  Port=13
  VTQD_TqSourceFr_enum : Inport  Port=14
  VTQD_TqSourceRr_enum : Inport  Port=15
  VVMC_ActMaxSlideRate_pct : Inport  Port=16
  VTQD_RDCActive_enum : Inport  Port=17
  task_time_s : Inport  Port=18
  VINP_HSAActive_flg : Inport  Port=19
  VINP_RrRBCActive_flg : Inport  Port=20
  VINP_FrRBCActive_flg : Inport  Port=21
  VVMC_ADASActive_flg : Inport  Port=22
  VTQD_APSReq_enum : Inport  Port=23
  VINP_AVHActive_flg : Inport  Port=24
  VVMC_APSSpeedCMD_kph : Inport  Port=25
  VVMC_APSActive_flg : Inport  Port=26
  VINP_FrEDURealTMTq_Nm : Inport  Port=27
  VINP_RrEDURealTMTq_Nm : Inport  Port=28
  VINP_ACCVehHoldReq_flg : Inport  Port=29
  VVMC_APSReq_enum : Inport  Port=30
  VVMC_LongAcc_Gps : Inport  Port=31
  VVMC_EstSlope_Deg : Inport  Port=32
  VINP_SCPSystemMode_enum : Inport  Port=33
  VPMM_PwrSta_enum : Inport  Port=34
  VINP_SWCResUpSta_flg : Inport  Port=35
  VINP_BrkPedalPos_pct : Inport  Port=36
  VTQR_NoABSFEDUWhlTqReq_Nm : Inport  Port=37
  VTQR_NoABSREDUWhlTqReq_Nm : Inport  Port=38
  VTQD_APSReqTimer_s : Inport  Port=39
  VINP_FrPTCSActive_flg : Inport  Port=40
  VINP_RrPTCSActive_flg : Inport  Port=41
  VINP_ADASACCSta_enum : Inport  Port=42
  VINP_EPBSta_enum : Inport  Port=43
  VTQD_OPDHoldEnRel_flg : Inport  Port=44
  VINP_SASAngle_Deg : Inport  Port=45
  VINP_YawRate_degps : Inport  Port=46
  VVMC_ActStESCYaw_degps : Inport  Port=47
  VVMC_CAASActive_flg : Inport  Port=48
  VVMC_ACCOvrdMemTq_Nm : Inport  Port=49
  VVMC_LastADASWhlTqReq_Nm : Inport  Port=50
  VTQD_OPDHoldActRelTq_Nm : Inport  Port=51
  BOS : Subsystem
  Creep : Subsystem
  DriverTqCoordination : Subsystem
  PedalMapWhlTq : Subsystem
  RollingRegenJudge : Subsystem
  VTQD_DriverWhlTqDem_Nm : Outport
  VTQD_RollRegenEnable_flg : Outport  Port=2
  VTQD_EVDriveModeValid_flg : Outport  Port=3
  VTQD_CreepEnable_flg : Outport  Port=4
  VTQD_LoSpdBrkCtrl_flg : Outport  Port=5
  VTQD_BOSEnable_flg : Outport  Port=6
  VTQD_OPDOn2Off_flg : Outport  Port=7
  VTQD_PreLoadHold_flg : Outport  Port=8
  VTQD_PreLoadPreEn_flg : Outport  Port=9
  VTQD_CreepPrLoadEnable_flg : Outport  Port=10
  VTQD_RegenTqLimitEn_flg : Outport  Port=11
  VTQD_VehActSpd_kph : Outport  Port=12
  VTQD_CreepBaseTqD_Nm : Outport  Port=13
  wires:
  VTQD_BrkSwSta_flg/1 -> [VTQD_BrkSwSta_flg]
  VTQD_ActBPSPosn_pct/1 -> [VTQD_ActBPSPosn_pct]
  VTQD_RegenMode_enum/1 -> [VTQD_RegenMode_enum]
  VINP_VehSpeed_kph/1 -> [VINP_VehSpeed_kph]
  "VTQD_CreepON_flg "/1 -> [VTQD_CreepON_flg]
  PedalMapWhlTq/1(VTQD_PedalMapWhlTq_Nm) -> [VTQD_PedalMapWhlTq_Nm]
  VTQD_LimpHomeAct_flg/1 -> [VTQD_LimpHomeAct_flg]
  VTQD_TqTargetShaftSpd_rpm/1 -> [VTQD_TqTargetShaftSpd_rpm]
  VTQD_EVDriveMode_enum/1 -> [VTQD_EVDriveMode_enum]
  VTQD_ActAPSPosn_pct/1 -> [VTQD_ActAPSPosn_pct]
  VTQD_GearActualPosn_enum/1 -> [VTQD_GearActualPosn_enum]
  VDHP_LowIdleAccPedal_flg/1 -> [VTQD_LowIdleAccPedal_flg]
  BOS/2(VTQD_BOSTq_Nm) -> [VTQD_BOSTq_Nm]
  BOS/1(VTQD_BOSEnable_flg) -> [VTQD_BOSEnable_flg], VTQD_BOSEnable_flg/1
  [VTQD_ActBPSPosn_pct] -> BOS/1(VTQD_ActBPSPosn_pct)
  [VTQD_TqTargetShaftSpd_rpm] -> BOS/2(VTQD_TqTargetShaftSpd_rpm)
  RollingRegenJudge/1(VTQD_RollRegenEnable_flg) -> VTQD_RollRegenEnable_flg/1, [VTQD_RollRegenEnable_flg]
  RollingRegenJudge/2(VTQD_RollingShaftSpd_rpm) -> [VTQD_RollingShaftSpd_rpm]
  VTQD_RollRegenDisableReq_flg/1 -> [VTQD_RollRegenDisableReq_flg]
  PedalMapWhlTq/2(VTQD_EVDriveModeValid_flg) -> VTQD_EVDriveModeValid_flg/1
  VTQD_TMRotateDirction_enum/1 -> [VTQD_TMRotateDirction_enum]
  [VTQD_GearActualPosn_enum] -> PedalMapWhlTq/1(VTQD_GearActualPosn_enum)
  [VTQD_LimpHomeAct_flg] -> PedalMapWhlTq/4(VTQD_LimpHomeAct_flg)
  [VTQD_ActAPSPosn_pct] -> PedalMapWhlTq/2(VTQD_ActAPSPosn_pct)
  [VTQD_TqTargetShaftSpd_rpm] -> PedalMapWhlTq/3(VTQD_TqTargetShaftSpd_rpm)
  [VTQD_RollRegenEnable_flg] -> PedalMapWhlTq/7(VTQD_RollRegenEnable_flg)
  [VTQD_RollingShaftSpd_rpm] -> PedalMapWhlTq/8(VTQD_RollingShaftSpd_rpm)
  [VTQD_RegenMode_enum] -> PedalMapWhlTq/6(VTQD_RegenMode_enum)
  [VTQD_EVDriveMode_enum] -> PedalMapWhlTq/5(VTQD_EVDriveMode_enum)
  [VTQD_TqSourceRr_enum] -> RollingRegenJudge/6(VTQD_TqSourceRr_enum)
  [VINP_VehSpeed_kph] -> RollingRegenJudge/2(VINP_VehSpd_kph)
  [VTQD_TqTargetShaftSpd_rpm] -> RollingRegenJudge/3(VTQD_TqTargetShaftSpd_rpm)
  [VTQD_TqSourceFr_enum] -> RollingRegenJudge/5(VTQD_TqSourceFr_enum)
  [VTQD_CreepEnable_flg] -> RollingRegenJudge/7(VTQD_CreepEnable_flg)
  [VTQD_LowIdleAccPedal_flg] -> RollingRegenJudge/1(VDHP_LowIdleAccPedal_flg)
  VTQD_TqSourceFr_enum/1 -> [VTQD_TqSourceFr_enum]
  VTQD_TqSourceRr_enum/1 -> [VTQD_TqSourceRr_enum]
  VVMC_ActMaxSlideRate_pct/1 -> [VVMC_ActMaxSlideRate_pct]
  VTQD_RDCActive_enum/1 -> [VTQD_RDCActive_enum]
  task_time_s/1 -> [task_time_s]
  [VTQD_RollRegenDisableReq_flg] -> RollingRegenJudge/4(VTQD_RollRegenDisableReq_flg)
  [VINP_VehSpeed_kph] -> DriverTqCoordination/7(VINP_VehSpeed_kph)
  [task_time_s] -> DriverTqCoordination/12(task_time_s)
  [VTQD_LowIdleAccPedal_flg] -> DriverTqCoordination/10(VTQD_LowIdleAccPedal_flg)
  [VTQD_GearActualPosn_enum] -> DriverTqCoordination/11(VTQD_GearActualPosn_enum)
  [VTQD_CreepPrLoadEnable_flg] -> DriverTqCoordination/2(VTQD_CreepPrLoadEnable_flg)
  [VTQD_PedalMapWhlTq_Nm] -> DriverTqCoordination/1(VTQD_PedalMapWhlTq_Nm)
  [VTQD_ActBPSPosn_pct] -> DriverTqCoordination/9(VTQD_ActBPSPosn_pct)
  [VTQD_BOSEnable_flg] -> DriverTqCoordination/4(VTQD_BOSEnable_flg)
  [VTQD_CreepWhlTqDem_Nm] -> DriverTqCoordination/3(VTQD_CreepWhlTqDem_Nm)
  [VTQD_BrkSwSta_flg] -> DriverTqCoordination/8(VTQD_BrkSwSta_flg)
  DriverTqCoordination/2(VTQD_LoSpdBrkCtrl_flg) -> [VTQD_LoSpdBrkCtrl_flg], VTQD_LoSpdBrkCtrl_flg/1
  DriverTqCoordination/1(VTQD_DriverWhlTqDem_Nm) -> VTQD_DriverWhlTqDem_Nm/1
  [VINP_RrRBCActive_flg] -> Creep/9(VINP_RrRBCActive_flg)
  [VINP_FrRBCActive_flg] -> Creep/10(VINP_FrRBCActive_flg)
  [VINP_VehSpeed_kph] -> Creep/4(VINP_VehSpeed_kph)
  [VTQD_ActBPSPosn_pct] -> Creep/7(VTQD_ActBPSPosn_pct)
  [VTQD_TMRotateDirction_enum] -> Creep/5(VTQD_TMRotateDirction_enum)
  [VTQD_CreepON_flg] -> Creep/1(VTQD_CreepON_flg)
  [VTQD_LowIdleAccPedal_flg] -> Creep/3(VTQD_LowIdleAccPedal_flg)
  [VTQD_APSReq_enum] -> Creep/15(VTQD_APSReq_enum)
  [VVMC_APSActive_flg] -> Creep/17(VVMC_APSActive_flg)
  [VTQD_RegenMode_enum] -> Creep/6(VTQD_RegenMode_enum)
  [VINP_AVHActive_flg] -> Creep/14(VINP_AVHActive_flg)
  [VVMC_APSSpeedCMD_kph] -> Creep/16(VVMC_APSSpeedCMD_kph)
  [VTQD_PedalMapWhlTq_Nm] -> Creep/8(VTQD_PedalMapWhlTq_Nm)
  [VTQD_GearActualPosn_enum] -> Creep/2(VTQD_GearActualPosn_enum)
  [VVMC_ADASActive_flg] -> Creep/11(VVMC_ADASActive_flg)
  [task_time_s] -> Creep/12(task_time_s)
  [VTQD_LoSpdBrkCtrl_flg] -> Creep/13(VTQD_LoSpdBrkCtrl_flg)
  Creep/1(VTQD_CreepEnable_flg) -> [VTQD_CreepEnable_flg], VTQD_CreepEnable_flg/1
  Creep/2(VTQD_CreepWhlTqDem_Nm) -> [VTQD_CreepWhlTqDem_Nm]  "VTQD_CreepWhlTqDem_Nm"
  Creep/3(VTQD_CreepPrLoadEnable_flg) -> VTQD_CreepPrLoadEnable_flg/1, [VTQD_CreepPrLoadEnable_flg]
  VVMC_APSActive_flg/1 -> [VVMC_APSActive_flg]
  VTQD_APSReq_enum/1 -> [VTQD_APSReq_enum]
  VVMC_ADASActive_flg/1 -> [VVMC_ADASActive_flg]
  VINP_AVHActive_flg/1 -> [VINP_AVHActive_flg]
  VVMC_APSSpeedCMD_kph/1 -> [VVMC_APSSpeedCMD_kph]
  VINP_FrRBCActive_flg/1 -> [VINP_FrRBCActive_flg]
  VINP_RrRBCActive_flg/1 -> [VINP_RrRBCActive_flg]
  VINP_HSAActive_flg/1 -> [VINP_HSAActive_flg]
  [VTQD_RollRegenDisableReq_flg] -> PedalMapWhlTq/9(VTQD_RollRegenDisableReq_flg)
  [VINP_HSAActive_flg] -> PedalMapWhlTq/10(VINP_HSAActive_flg)
  Creep/4(VTQD_OPDOn2Off_flg) -> VTQD_OPDOn2Off_flg/1
  VINP_RrEDURealTMTq_Nm/1 -> [VINP_RrEDURealTMTq_Nm]
  VINP_FrEDURealTMTq_Nm/1 -> [VINP_FrEDURealTMTq_Nm]
  [VINP_FrEDURealTMTq_Nm] -> DriverTqCoordination/13(VINP_FrEDURealTMTq_Nm)
  [VINP_RrEDURealTMTq_Nm] -> DriverTqCoordination/14(VINP_RrEDURealTMTq_Nm)
  DriverTqCoordination/3(VTQD_PreLoadHold_flg) -> VTQD_PreLoadHold_flg/1
  [VVMC_ADASActive_flg] -> PedalMapWhlTq/11(VVMC_ADASActive_flg)
  [VTQD_RDCActive_enum] -> Creep/18(VTQD_RDCActive_enum)
  VINP_ACCVehHoldReq_flg/1 -> [VINP_ACCVehHoldReq_flg]
  VVMC_APSReq_enum/1 -> [VVMC_APSReq_enum]
  [VVMC_APSReq_enum] -> Creep/19(VVMC_APSReq_enum)
  [VVMC_APSActive_flg] -> DriverTqCoordination/15(VVMC_APSActive_flg)
  [VVMC_ADASActive_flg] -> DriverTqCoordination/16(VVMC_ADASActive_flg)
  [VINP_ACCVehHoldReq_flg] -> DriverTqCoordination/17(VINP_ACCVehHoldReq_flg)
  [VINP_RrEDURealTMTq_Nm] -> Creep/21(VINP_RrEDURealTMTq_Nm)
  [VINP_FrEDURealTMTq_Nm] -> Creep/20(" VINP_FrEDURealTMTq_Nm")
  Creep/5(VTQD_CreepProtTqEn_flg) -> [VTQD_CreepProtTqEn_flg]
  [VTQD_CreepProtTqEn_flg] -> DriverTqCoordination/18(VTQD_CreepProtTqEn_flg)
  [VVMC_ActMaxSlideRate_pct] -> PedalMapWhlTq/12(VVMC_ActMaxSlideRate_pct)
  VVMC_LongAcc_Gps/1 -> [VVMC_LongAcc_Gps]
  VVMC_EstSlope_Deg/1 -> [VVMC_EstSlope_Deg]
  [VVMC_LongAcc_Gps] -> PedalMapWhlTq/14(VVMC_LongAcc_Gps)
  [VVMC_EstSlope_Deg] -> PedalMapWhlTq/13(VVMC_EstSlope_Deg)
  PedalMapWhlTq/3(VTQD_RegenTqLimitEn_flg) -> VTQD_RegenTqLimitEn_flg/1
  DriverTqCoordination/4(VTQD_PreLoadPreEn_flg) -> [VTQD_PreLoadPreEn_flg], VTQD_PreLoadPreEn_flg/1
  [VTQD_PreLoadPreEn_flg] -> Creep/22(VTQD_PreLoadPreEn_flg)
  [VVMC_EstSlope_Deg] -> Creep/23(VVMC_EstSlope_Deg)
  [VPMM_PwrSta_enum] -> Creep/24(VPMM_PwrSta_enum)
  [VTQD_TqTargetShaftSpd_rpm] -> DriverTqCoordination/19(VTQD_TqTargetShaftSpd_rpm)
  [VINP_SCPSystemMode_enum] -> PedalMapWhlTq/15(VINP_SCPSystemMode_enum)
  [VPMM_PwrSta_enum] -> PedalMapWhlTq/16(VPMM_PwrSta_enum)
  [VINP_SWCResUpSta_flg] -> PedalMapWhlTq/17(VINP_SWCResUpSta_flg)
  [task_time_s] -> PedalMapWhlTq/18(task_time_s)
  [VINP_VehSpeed_kph] -> PedalMapWhlTq/19(VINP_VehSpeed_kph)
  [VTQD_CreepPrLoadEnable_flg] -> PedalMapWhlTq/20(VTQD_CreepPrLoadEnable_flg)
  [VINP_BrkPedalPos_pct] -> PedalMapWhlTq/21(VINP_BrkPedalPos_pct)
  [VTQR_NoABSREDUWhlTqReq_Nm] -> PedalMapWhlTq/22(VTQR_NoABSREDUWhlTqReq_Nm)
  [VTQR_NoABSFEDUWhlTqReq_Nm] -> PedalMapWhlTq/23(VTQR_NoABSFEDUWhlTqReq_Nm)
  [VINP_FrPTCSActive_flg] -> PedalMapWhlTq/24(VINP_FrPTCSActive_flg)
  [VINP_RrPTCSActive_flg] -> PedalMapWhlTq/25(VINP_RrPTCSActive_flg)
  [VINP_ADASACCSta_enum] -> PedalMapWhlTq/26(VINP_ADASACCSta_enum)
  [VTQD_LowIdleAccPedal_flg] -> PedalMapWhlTq/27(VTQD_LowIdleAccPedal_flg)
  [VTQD_BrkSwSta_flg] -> PedalMapWhlTq/28(VTQD_BrkSwSta_flg)
  [VTQD_TqTargetShaftSpd_rpm] -> Creep/25(VTQD_TqTargetShaftSpd_rpm)
  [VTQD_APSReqTimer_s] -> Creep/26(VTQD_APSReqTimer_s)
  [VINP_EPBSta_enum] -> Creep/27(VINP_EPBSta_enum)
  Creep/6(VTQD_VehActSpd_kph) -> VTQD_VehActSpd_kph/1, [VTQD_VehActSpd_kph]
  VINP_EPBSta_enum/1 -> [VINP_EPBSta_enum]
  VINP_RrPTCSActive_flg/1 -> [VINP_RrPTCSActive_flg]
  VINP_SCPSystemMode_enum/1 -> [VINP_SCPSystemMode_enum]
  VINP_BrkPedalPos_pct/1 -> [VINP_BrkPedalPos_pct]
  VINP_FrPTCSActive_flg/1 -> [VINP_FrPTCSActive_flg]
  VTQD_APSReqTimer_s/1 -> [VTQD_APSReqTimer_s]
  VTQR_NoABSFEDUWhlTqReq_Nm/1 -> [VTQR_NoABSFEDUWhlTqReq_Nm]
  VINP_ADASACCSta_enum/1 -> [VINP_ADASACCSta_enum]
  VTQR_NoABSREDUWhlTqReq_Nm/1 -> [VTQR_NoABSREDUWhlTqReq_Nm]
  VINP_SWCResUpSta_flg/1 -> [VINP_SWCResUpSta_flg]
  VPMM_PwrSta_enum/1 -> [VPMM_PwrSta_enum]
  [VTQD_PedalMapWhlTq_Nm] -> BOS/4(VTQD_PedalMapWhlTq_Nm)
  [VTQD_VehActSpd_kph] -> BOS/3(VTQD_VehActSpd_kph)
  Creep/7(VTQD_CreepBaseTqD_Nm) -> VTQD_CreepBaseTqD_Nm/1, [VTQD_CreepBaseTqD_Nm]
  Creep/8(VTQD_CreepBaseTqR_Nm) -> [VTQD_CreepBaseTqR_Nm]
  [VTQD_BOSTq_Nm] -> DriverTqCoordination/5(VTQD_BOSTq_Nm)
  [VTQD_CreepBaseTqR_Nm] -> BOS/5(VTQD_CreepBaseTqR_Nm)
  [VTQD_CreepBaseTqD_Nm] -> BOS/6(VTQD_CreepBaseTqD_Nm)
  [VTQD_GearActualPosn_enum] -> BOS/7(VTQD_GearActualPosn_enum)
  VTQD_OPDHoldEnRel_flg/1 -> [VTQD_OPDHoldEnRel_flg]
  [VTQD_OPDHoldEnRel_flg] -> Creep/28(VTQD_OPDHoldEnRel_flg)
  [VVMC_APSActive_flg] -> BOS/8(VVMC_APSActive_flg)
  [VTQD_VehActSpd_kph] -> DriverTqCoordination/20(VTQD_VehActSpd_kph)
  [VTQD_ActAPSPosn_pct] -> Creep/29(VTQD_ActAPSPosn_pct)
  [VTQD_APSReqTimer_s] -> DriverTqCoordination/21(VTQD_APSReqTimer_s)
  [VTQD_CreepEnable_flg] -> DriverTqCoordination/22(VTQD_CreepEnable_flg)
  [VTQD_OPDHoldEnRel_flg] -> PedalMapWhlTq/29(VTQD_OPDHoldEnRel_flg)
  [VINP_SASAngle_Deg] -> PedalMapWhlTq/30(VINP_SASAngle_Deg)
  [VINP_YawRate_degps] -> PedalMapWhlTq/31(VINP_YawRate_degps)
  [VVMC_ActStESCYaw_degps] -> PedalMapWhlTq/32(VVMC_ActStESCYaw_degps)
  VINP_SASAngle_Deg/1 -> [VINP_SASAngle_Deg]
  VINP_YawRate_degps/1 -> [VINP_YawRate_degps]
  VVMC_ActStESCYaw_degps/1 -> [VVMC_ActStESCYaw_degps]
  VVMC_CAASActive_flg/1 -> [VVMC_CAASActive_flg]
  [VVMC_CAASActive_flg] -> Creep/30(VVMC_CAASActive_flg)
  [VVMC_LongAcc_Gps] -> DriverTqCoordination/6(VVMC_LongAcc_Gps)
  [VTQD_APSReqTimer_s] -> PedalMapWhlTq/33(VTQD_APSReqTimer_s)
  [VTQD_LowIdleAccPedal_flg] -> BOS/9(VTQD_LowIdleAccPedal_flg)
  [VVMC_ACCOvrdMemTq_Nm] -> PedalMapWhlTq/34(VVMC_ACCOvrdMemTq_Nm)
  VVMC_ACCOvrdMemTq_Nm/1 -> [VVMC_ACCOvrdMemTq_Nm]
  VVMC_LastADASWhlTqReq_Nm/1 -> PedalMapWhlTq/35(VVMC_LastADASWhlTqReq_Nm)
  [VTQD_OPDHoldActRelTq_Nm] -> PedalMapWhlTq/36(VTQD_OPDHoldActRelTq_Nm)
  [VTQD_VehActSpd_kph] -> PedalMapWhlTq/37(VTQD_VehActSpd_kph)
  Creep/9(VTQD_HighBPSPosn_flg) -> [VTQD_HighBPSPosn_flg]
  [VTQD_HighBPSPosn_flg] -> BOS/10(VTQD_HighBPSPosn_flg)
  [VTQD_BrkSwSta_flg] -> BOS/11(VTQD_BrkSwSta_flg)
  VTQD_OPDHoldActRelTq_Nm/1 -> [VTQD_OPDHoldActRelTq_Nm]
